simulink model "noise_bandwidth_simulink"  (R2016b)
settings: Solver=VariableStepDiscrete  StartTime=0.0  StopTime=10  RelTol=1e-3
values from neighbouring files (symbols this model uses):
  lam = 1-zp    [noise_bandwidth.m]
  N0 = sig2a/SNR    (= 0.1)    [MSE_matlab2.m]    (also in adaptive_equalization.m = 0.0316227766017; noise_bandwidth.m = 2)
  zp = 1-2^(-n)    [noise_bandwidth.m]
libraries: dspstat3 x2, dspspect3 x1, dspsrcs4 x1, dspmathops x1
settings Model: Creator=Shu  LastModifiedBy=Shu
settings DataIOCC: LimitDataPoints=on  SaveOutput=off  SaveTime=off
settings OptimizationCC: BooleanDataType=off  DefaultParameterBehavior=Inlined  LocalBlockOutputs=off  LifeSpan=inf
settings DebuggingCC: AlgebraicLoopMsg=error  SingleTaskRateTransMsg=error  AllowSymbolicDim=off  SFUnexpectedBacktrackingDiag=warning  SFNoUnconditionalDefaultTransitionDiag=warning  SFExecutionAtInitializationDiag=none
settings GRTTargetCC: TargetLangStandard=C89/C90 (ANSI)  GeneratePreprocessorConditionals=Disable all
settings ConfigComp: CovMetricSettings=dw  CovHtmlReporting=on  CovSaveCumulativeToWorkspaceVar=on  CovSaveSingleToWorkspaceVar=on  CovExternalEMLEnable=off  CovSFcnEnable=off

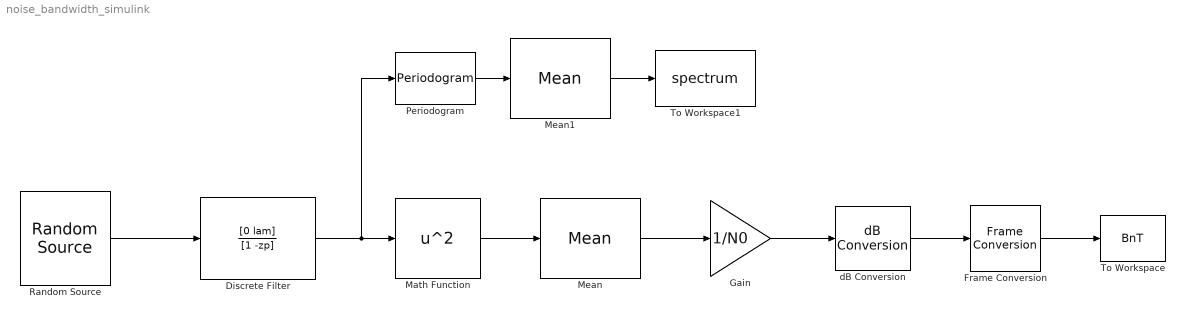
== system noise_bandwidth_simulink ==
  Discrete Filter : DiscreteFilter  Numerator=[0 lam]  Denominator=[1 -zp]
  Frame Conversion : FrameConversion  InheritSamplingMode=off  OutFrame=Sample-based
  Gain : Gain  Gain=1/N0
  Math Function : Math  Operator=square  SaturateOnIntegerOverflow=on
  Mean : dspstat3/Mean  run=on  reset_popup=None  directionMode=Each column  dimension=1  roiEnable=off  roiType=Rectangles  roiPortion=Entire ROI  roiOutput=Individual statistics for each ROI  roiFlag=off  outputDataTypeStr=Inherit: Same as accumulator  outputLastDataTypeStr=Inherit: Same as accumulator  outputMin=[]  outputMax=[]  roundingMode=Floor  overflowMode=off
  Mean1 : dspstat3/Mean  run=on  reset_popup=None  directionMode=Each column  dimension=1  roiEnable=off  roiType=Rectangles  roiPortion=Entire ROI  roiOutput=Individual statistics for each ROI  roiFlag=off  outputDataTypeStr=Inherit: Same as accumulator  outputLastDataTypeStr=Inherit: Same as accumulator  outputMin=[]  outputMax=[]  roundingMode=Floor  overflowMode=off
  Periodogram : dspspect3/Periodogram  measurement=Power spectral density  wintype=Hamming  Rs=50  beta=5  winsamp=Symmetric  FFTImplementation=Auto  inheritFFT=off  fftsize=256  navg=4  inheritTs=on  Ts=1
  Random Source : dspsrcs4/Random Source  SrcType=Gaussian  NormMethod=Ziggurat  CltLength=12  MinVal=0  MaxVal=1  MeanVal=0  VarVal=N0  RepMode=Not repeatable  rawSeed=1  IsInherit=off  SampMode=Discrete  SampTime=1  SampFrame=framelength  DataType=Double  OutComplex=Real  OutputFrames=off
  To Workspace : ToWorkspace  VariableName=BnT  SampleTime=-1
      settings: MaxDataPoints=1
  To Workspace1 : ToWorkspace  VariableName=spectrum  SampleTime=-1
      settings: MaxDataPoints=1
  dB Conversion : dspmathops/dB Conversion  dBtype=dB  intype=Power  R=1  fuzz=off
  wires:
  Random Source/1 -> Discrete Filter/1
  Discrete Filter/1 -> Periodogram/1, Math Function/1
  Math Function/1 -> Mean/1
  Mean/1 -> Gain/1
  Frame Conversion/1 -> To Workspace/1
  dB Conversion/1 -> Frame Conversion/1
  Gain/1 -> dB Conversion/1
  Periodogram/1 -> Mean1/1
  Mean1/1 -> To Workspace1/1
